simulink model "SkywalkerX8_ClassicalControl"  (R2018a)
settings: Solver=VariableStepAuto  StartTime=0.0  StopTime=10.0  RelTol=1e-3
libraries: aerolibatmos2 x1
settings Model: Creator=David  LastModifiedBy=David

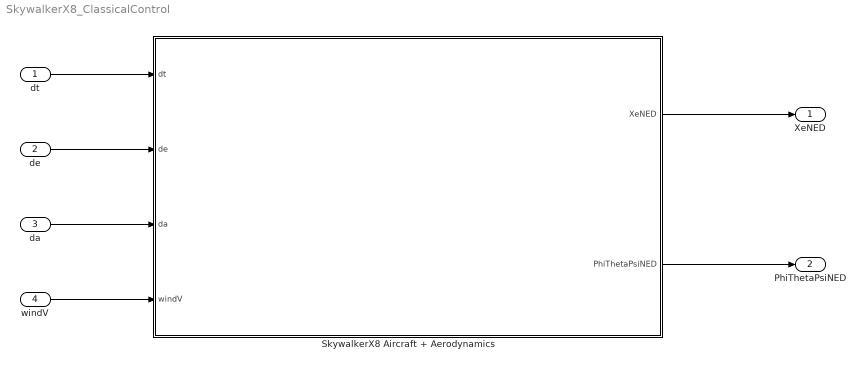
== system SkywalkerX8_ClassicalControl ==
  dt : Inport
  de : Inport  Port=2
  da : Inport  Port=3
  windV : Inport  Port=4
  SkywalkerX8 Aircraft + Aerodynamics : Subsystem
      mask Display:
      | image('x8SkySunset.png', 'center')
      | 
      | port_label('input', 1, '\delta_t (Unitless)', 'texmode', 'on')
      | port_label('input', 2, '\delta_e (rad)', 'texmode', 'on')
      | port_label('input', 3, '\delta_a (rad)', 'texmode', 'on')
      | port_label('input', 4, '{\bf V_w^b} (m/s)', 'texmode', 'on')
      | 
      | port_label('output', 1, '{\bf X_e_{NED}} (m)', 'texmode', 'on')
      | port_label('output', 2, '(\phi \theta \psi)_{NED} (rad)', 'texmode', 'on')
  XeNED : Outport
  PhiThetaPsiNED : Outport  Port=2
  wires:
  da/1 -> SkywalkerX8 Aircraft + Aerodynamics/3(da)
  dt/1 -> SkywalkerX8 Aircraft + Aerodynamics/1(dt)
  windV/1 -> SkywalkerX8 Aircraft + Aerodynamics/4(windV)
  de/1 -> SkywalkerX8 Aircraft + Aerodynamics/2(de)
  SkywalkerX8 Aircraft + Aerodynamics/1(XeNED) -> XeNED/1
  SkywalkerX8 Aircraft + Aerodynamics/2(PhiThetaPsiNED) -> PhiThetaPsiNED/1

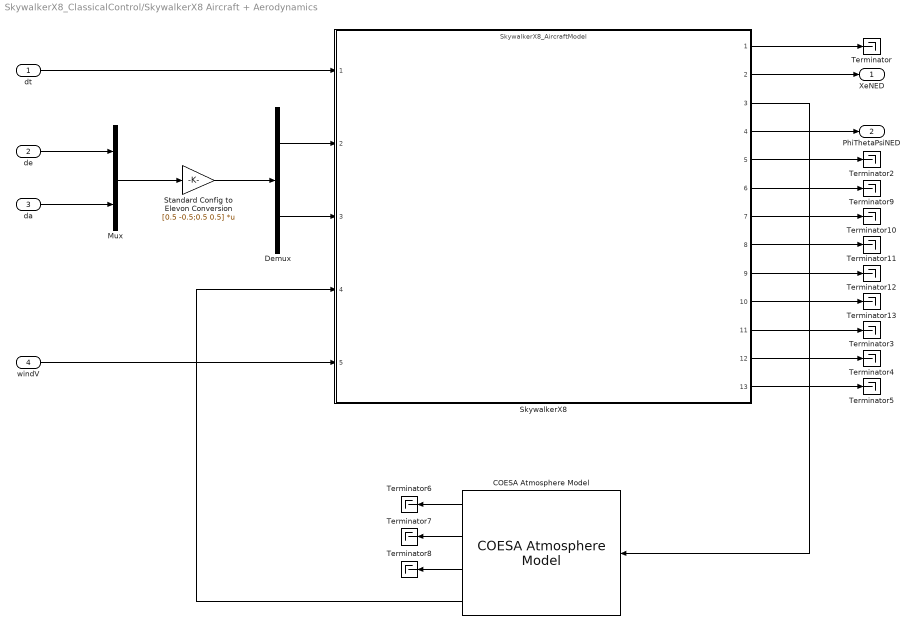
== system SkywalkerX8_ClassicalControl/SkywalkerX8 Aircraft + Aerodynamics ==
  dt : Inport
  de : Inport  Port=2
  da : Inport  Port=3
  windV : Inport  Port=4
  COESA Atmosphere Model : aerolibatmos2/COESA Atmosphere Model  units=Metric (MKS)  spec=1976 COESA-extended U.S. Standard Atmosphere  model=Profile  profile_var=High temperature  profile_percent=1%  profile_alt=5 km (16404 ft)  envelope_var=High temperature  envelope_percent=1%  action=None
  Demux : Demux  Outputs=2
  Mux : Mux  Inputs=2
  SkywalkerX8 : ModelReference  ModelNameDialog=SkywalkerX8_AircraftModel  ModelReferenceVersion=1.163
      mask Display:
      | image('C:\MATLAB\masters\icons\Skywalker Main Block Icon.png', 'center')
      | 
      | color('cyan')
      | 
      | port_label('input', 1, 'k_{motor} (Unitless)', 'texmode', 'on')
      | port_label('input', 2, '\delta_{er} (rad)', 'texmode', 'on')
      | port_label('input', 3, '\delta_{el} (rad)', 'texmode', 'on')
      | port_label('input', 4, '\rho (kg/m^3)', 'texmode', 'on')
      | port_label('input', 5, '{\bf V_w^b} (m/s)', 'texmode', 'on')
      | 
      | port_label('output', 1, '{\bf V_e} (m/s)', 'texmode', 'on')
      | port_label('output', 2, '{\bf X_e} (m)', 'texmode', 'on')
      | port_label('output', 3, 'Altitude (m)', 'texmode', 'on')
      | port_label('output', 4, '\phi \theta \psi (rad)', 'texmode', 'on')
      | port_label('output', 5, 'R_{inertial}^{body}', 'texmode', 'on')
      | port_label('output', 6, 'V_a (m/s)', 'texmode', 'on')
      | port_label('output', 7, 'alpha (rad)', 'texmode', 'on')
      | port_label('output', 8, 'beta (rad)', 'texmode', 'on')
      | port_label('output', 9, '{\bf V_b} (m/s)', 'texmode', 'on')
      | port_label('output', 10, '{\bf \omega_b} (rad/s)', 'texmode', 'on')
      | port_label('output', 11, '{\bf \delta\omega_b/\deltat} (rad/s^2)', 'texmode', 'on')
      | port_label('output', 12, '{\bf a_{body}} (m/s^2)', 'texmode', 'on')
      | port_label('output', 13, '{\bf a_{inertial}} (m/s^2)', 'texmode', 'on')
  Standard Config to Elevon Conversion : Gain  Gain=[0.5 -0.5;0.5 0.5]  Multiplication=Matrix(K*u)
  Terminator{,2..13} (13 alike) : Terminator
  XeNED : Outport
  PhiThetaPsiNED : Outport  Port=2
  wires:
  SkywalkerX8/12 -> Terminator4/1
  COESA Atmosphere Model/2 -> Terminator7/1
  COESA Atmosphere Model/1 -> Terminator6/1
  Demux/2 -> SkywalkerX8/3
  SkywalkerX8/13 -> Terminator5/1
  COESA Atmosphere Model/3 -> Terminator8/1
  Mux/1 -> Standard Config to Elevon Conversion/1
  windV/1 -> SkywalkerX8/5
  SkywalkerX8/11 -> Terminator3/1
  SkywalkerX8/6 -> Terminator9/1
  COESA Atmosphere Model/4 -> SkywalkerX8/4
  SkywalkerX8/1 -> Terminator/1
  SkywalkerX8/5 -> Terminator2/1
  Standard Config to Elevon Conversion/1 -> Demux/1
  de/1 -> Mux/1
  Demux/1 -> SkywalkerX8/2
  SkywalkerX8/7 -> Terminator10/1
  dt/1 -> SkywalkerX8/1
  da/1 -> Mux/2
  SkywalkerX8/8 -> Terminator11/1
  SkywalkerX8/3 -> COESA Atmosphere Model/1
  SkywalkerX8/9 -> Terminator12/1
  SkywalkerX8/10 -> Terminator13/1
  SkywalkerX8/2 -> XeNED/1
  SkywalkerX8/4 -> PhiThetaPsiNED/1
